simulink model "modelo_experimental"  (R2018a)
settings: Solver=ode4  StartTime=0.0  StopTime=1.0  FixedStep=0.001  RelTol=1e-3  EnableMultiTasking=on
values from neighbouring files (symbols this model uses):
  A = [0  1; 0  -12.380613988]    [params_ts03_mp10.mat]    (also in setup_pi_control.m = [0 1; 0 -a])
  B = [0 1.46056704108]    [params_ts03_mp10.mat]    (also in setup_pi_control.m = [0; b])
  C = [1 0]    [params_ts03_mp10.mat]    (also in setup_pi_control.m)
  D = 0    [params_ts03_mp10.mat]    (also in setup_pi_control.m)
  Gaa = 1    [params_ts03_mp10.mat]    (also in setup_pi_control.m = G(1, 1))
  Gab = 0.00940574437646    [params_ts03_mp10.mat]    (also in setup_pi_control.m = G(1, 2))
  Gba = 0    [params_ts03_mp10.mat]    (also in setup_pi_control.m = G(2, 1))
  Gbb = 0.883551109605    [params_ts03_mp10.mat]    (also in setup_pi_control.m = G(2, 2))
  Ha = 0.0294443454095    [params_ts03_mp10.mat]    (also in setup_pi_control.m = H(1, 1))
  Hb = 5.76984249791    [params_ts03_mp10.mat]    (also in setup_pi_control.m = H(2, 1))
  K1 = 0.770639270936    [params_ts03_mp10.mat]    (also in setup_pi_control.m = K1_bar)
  K2 = [4.4341828223 0.174846170282]    [params_ts03_mp10.mat]    (also in setup_pi_control.m = K2_bar/P)
  Ke = 83.305592651    [params_ts03_mp10.mat]    (also in setup_pi_control.m = (Gbb - polo_min)/Gab)
settings Model: Creator=mtsousa  LastModifiedBy=mtsousa

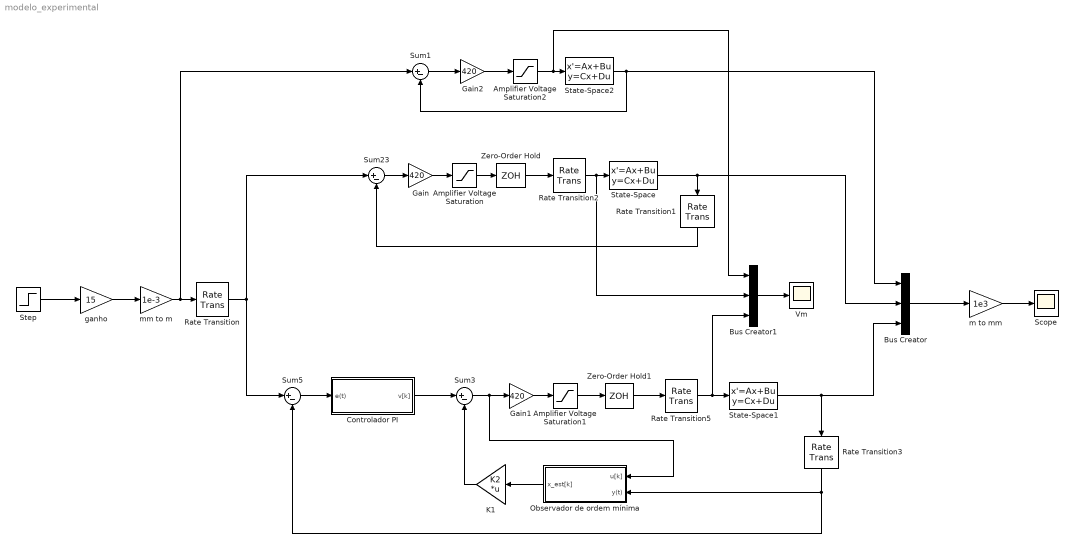
== system modelo_experimental ==
  Amplifier Voltage Saturation : Saturate  UpperLimit=12  LowerLimit=-12
  Amplifier Voltage Saturation1 : Saturate  UpperLimit=12  LowerLimit=-12
  Amplifier Voltage Saturation2 : Saturate  UpperLimit=12  LowerLimit=-12
  Bus Creator : BusCreator  Inputs=3
  Bus Creator1 : BusCreator  Inputs=3
  Controlador PI : Subsystem
  Gain : Gain  Gain=420
  Gain1 : Gain  Gain=420
  Gain2 : Gain  Gain=420
  K1 : Gain  Gain=K2  Multiplication=Matrix(K*u)
  Observador de ordem mínima : Subsystem
  Rate Transition : RateTransition  Deterministic=off  OutPortSampleTime=T
  Rate Transition1 : RateTransition  Deterministic=off  OutPortSampleTime=T
  Rate Transition2 : RateTransition  Deterministic=off  OutPortSampleTimeMultiple=0.001  OutPortSampleTime=0.001
  Rate Transition3 : RateTransition  Deterministic=off  OutPortSampleTime=T
  Rate Transition5 : RateTransition  Deterministic=off  OutPortSampleTime=0.001
  Scope : Scope
  State-Space : StateSpace  A=A  B=B  C=C  D=D  InitialCondition=0
  State-Space1 : StateSpace  A=A  B=B  C=C  D=D  InitialCondition=0
  State-Space2 : StateSpace  A=A  B=B  C=C  D=D  InitialCondition=0
  Step : Step  Time=0  SampleTime=0
  Sum{1,3,5,23} (4 alike) : Sum  Inputs=|+-
  Vm : Scope
  Zero-Order Hold : ZeroOrderHold  SampleTime=-1
  Zero-Order Hold1 : ZeroOrderHold  SampleTime=-1
  ganho : Gain  Gain=15  SaturateOnIntegerOverflow=on  OutDataTypeStr=Inherit: Same as input  ParamDataTypeStr=Inherit: Same as input
  m to mm : Gain  Gain=1e3  SaturateOnIntegerOverflow=on  OutDataTypeStr=Inherit: Same as input  ParamDataTypeStr=Inherit: Same as input
  mm to m : Gain  Gain=1e-3  SaturateOnIntegerOverflow=on  OutDataTypeStr=Inherit: Same as input  ParamDataTypeStr=Inherit: Same as input
  wires:
  Sum23/1 -> Gain/1
  Amplifier Voltage Saturation/1 -> Zero-Order Hold/1
  Zero-Order Hold/1 -> Rate Transition2/1
  Gain/1 -> Amplifier Voltage Saturation/1
  ganho/1 -> mm to m/1
  Step/1 -> ganho/1
  m to mm/1 -> Scope/1
  Bus Creator1/1 -> Vm/1
  Bus Creator/1 -> m to mm/1
  Rate Transition2/1 -> Bus Creator1/2, State-Space/1
  State-Space/1 -> Bus Creator/2, Rate Transition1/1
  Rate Transition3/1 -> Sum5/2, Observador de ordem mínima/2(y(t))
  State-Space1/1 -> Bus Creator/3, Rate Transition3/1
  Sum5/1 -> Controlador PI/1(e(t))
  Rate Transition5/1 -> Bus Creator1/3, State-Space1/1
  Zero-Order Hold1/1 -> Rate Transition5/1
  Amplifier Voltage Saturation1/1 -> Zero-Order Hold1/1
  Observador de ordem mínima/1(x_est[k]) -> K1/1
  Sum3/1 -> Gain1/1, Observador de ordem mínima/1(u[k])
  Gain1/1 -> Amplifier Voltage Saturation1/1
  Controlador PI/1(v[k]) -> Sum3/1
  K1/1 -> Sum3/2
  Rate Transition1/1 -> Sum23/2
  Rate Transition/1 -> Sum5/1, Sum23/1
  Gain2/1 -> Amplifier Voltage Saturation2/1
  Sum1/1 -> Gain2/1
  State-Space2/1 -> Bus Creator/1, Sum1/2
  Amplifier Voltage Saturation2/1 -> Bus Creator1/1, State-Space2/1
  mm to m/1 -> Sum1/1, Rate Transition/1

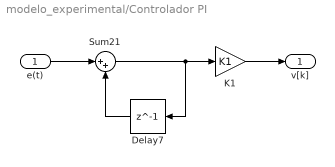
== system modelo_experimental/Controlador PI ==
  e(t) : Inport
  Delay7 : Delay  DelayLength=1
  K1 : Gain  Gain=K1
  Sum21 : Sum  Inputs=|++
  v[k] : Outport
  wires:
  Delay7/1 -> Sum21/2
  Sum21/1 -> Delay7/1, K1/1
  e(t)/1 -> Sum21/1
  K1/1 -> v[k]/1

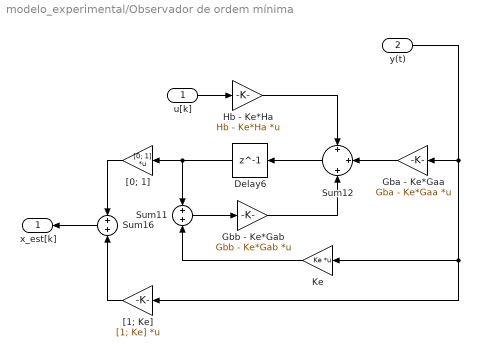
== system modelo_experimental/Observador de ordem mínima ==
  u[k] : Inport
  y(t) : Inport  Port=2
  Delay6 : Delay  DelayLength=1
  Gba - Ke*Gaa : Gain  Gain=Gba - Ke*Gaa  Multiplication=Matrix(K*u)
  Gbb - Ke*Gab : Gain  Gain=Gbb - Ke*Gab  Multiplication=Matrix(K*u)
  Hb - Ke*Ha : Gain  Gain=Hb - Ke*Ha  Multiplication=Matrix(K*u)
  Ke : Gain  Gain=Ke  Multiplication=Matrix(K*u)
  Sum11 : Sum  Inputs=+|+
  Sum12 : Sum  Inputs=+|+|+
  Sum16 : Sum  Inputs=+|+
  "[0; 1]" : Gain  Gain=[0; 1]  Multiplication=Matrix(K*u)
  "[1; Ke]" : Gain  Gain=[1; Ke]  Multiplication=Matrix(K*u)
  x_est[k] : Outport  PortDimensions=[2; 1]
  wires:
  Sum12/1 -> Delay6/1
  Delay6/1 -> "[0; 1]"/1, Sum11/1
  "[0; 1]"/1 -> Sum16/1
  Hb - Ke*Ha/1 -> Sum12/1
  Sum11/1 -> Gbb - Ke*Gab/1
  Gbb - Ke*Gab/1 -> Sum12/3
  Ke/1 -> Sum11/2
  "[1; Ke]"/1 -> Sum16/2
  Gba - Ke*Gaa/1 -> Sum12/2
  u[k]/1 -> Hb - Ke*Ha/1
  Sum16/1 -> x_est[k]/1
  y(t)/1 -> "[1; Ke]"/1, Ke/1, Gba - Ke*Gaa/1
